simulink library "NelinSys"  (Simulink 2.20)
values from neighbouring files (symbols this model uses):
  v = menu('EXACT LINEARIZATION (demo simulations)',    'Exact linearization of SISO system',    'Exact linearization of MIMO system',    'System with unstable zero dynamics')    [demos_exakt.m]    (also in demos_fp.m = menu('PHASE PLANE ANALYSIS (demo simulations)',    '2nd-Orde; demos_gs.m = menu('GAIN SCHEDULING (demo simulations)',    'Input and out)
  x1 = x(j)    [fazrov_auton2.m]
  x2 = x(j+1)    [fazrov_auton2.m]    (also in fazrov_typ1.m = get_param(get_param(gcbh,'Parent'),'UserData'))
undefined symbols (not defined in the file or in its folder): sfunvxy
libraries: simulink x5
(part 1 of 2)

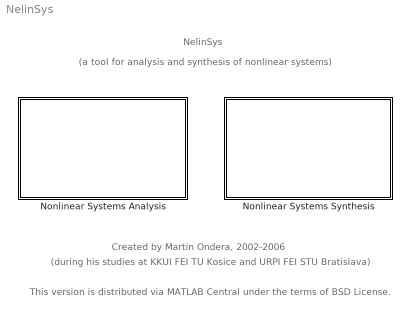
== system NelinSys ==
  note: (a tool for analysis and synthesis of nonlinear systems)
  note: NelinSys
  note: Created by Martin Ondera, 2002-2006
  note: (during his studies at KKUI FEI TU Kosice and URPI FEI STU Bratislava)
  note: This version is distributed via MATLAB Central under the terms of BSD License.
  Nonlinear Systems Analysis : Subsystem
      mask Type: Nonlinear Systems Analysis
      mask Display: disp('Analysis');
  Nonlinear Systems Synthesis : Subsystem
      mask Type: Nonlinear Systems Synthesis
      mask Display: disp('Synthesis');

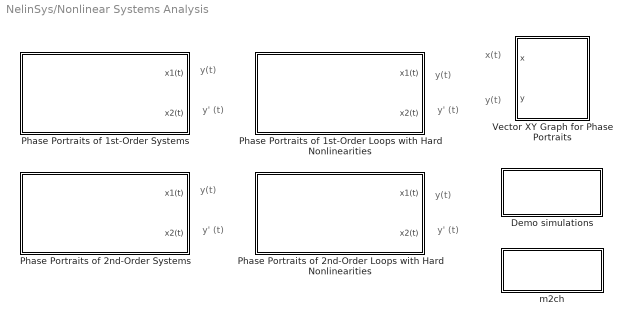
== system NelinSys/Nonlinear Systems Analysis ==
  note: y(t)
  note: y' (t)
  note: x(t)
  note: y(t)
  note: y(t)
  note: y' (t)
  note: y(t)
  note: y' (t)
  note: y(t)
  note: y' (t)
  Demo simulations : Subsystem
      settings: OpenFcn=demos_fp
      mask Display: disp('Phase Plane\nAnalysis')
  Phase Portraits of 1st-Order Loops with Hard Nonlinearities : Subsystem  mask(Phase-Plane Portrait of a 1st-Order Loop with a Hard Nonlinearity){num=0.01, den=[1 0.01], nelintyp=Relay with hysteresis, nelinpar=[-1 0 1 100], w=20, x10=[0 25]}
      mask prompts: num "Linear part - transfer function numerator:"; den "Linear part - transfer function denominator:"; nelintyp "Nonlinear part - nonlinearity type:"; nelinpar "Nonlinear part - parameters:"; w "Setpoint:"; x10 "Initial conditions: x1(0) = y(0) ="
      mask help:
      | Computation of a phase-plane portrait of a closed loop system consisting of an isolated hard nonlinearity and a linear part specified by a 1st-order transfer function.
      |
      | Block has two vector outputs, y = x1 (system output) and y' = x2 (derivative of the system output), i.e. horizontal and vertical coordinates of phase-plane trajectories corresponding to different initial conditions - the initial conditions themselves are specified by the vector x1(0) below.
      |
      | It is recommended to use the "Vector XY Graph for Phase Portraits" block to plot the portrait graphically, since the "XY Graph" block from Sinks library cannot handle vector inputs.
      |
      | For a detailed description of the block, click "Help" button.
      mask init:
      | if (length(den) ~= 2) | (length(num) ~= 1) | (den(1) == 0)
      |     error('Linear part must be a 1st-order system!');
      | end
      | 
      | if (nelintyp == 1) & (length(nelinpar) ~= 2)
      |     error('Invalid number of nonlinearity parameters!');
      | end
      | if (nelintyp > 1) & ((length(nelinpar) ~= 4) | nelinpar(1) > nelinpar(3))
      |     error('Invalid nonlinearity parameters!');
      | end
      | 
      | for k = 1:length(x10)
      |     if (w-x10(k)>nelinpar(1)) & (w-x10(k)<nelinpar(3))
      |         error(['Invalid initial conditions!']);
      |     end
      | end
      mask Help: web(fullfile(cd,'help','fazrov_typ1.html'));
      mask StyleString: edit,edit,popup(Ideal relay|Saturation|Relay with dead-zone|Relay with hysteresis),edit,edit,edit
      mask Display: disp('Phase Portraits of\n1st-Order Loops\nwith Hard Nonlinearities');
  Phase Portraits of 1st-Order Systems : Subsystem  mask(Phase-Plane Portrait of a 1st-Order Autonomous System){vRovnica=Dy-y^2+1=0, x10=[-10 0.9999 (1+1e-6)]}
      mask prompts: vRovnica "System differential equation: y' + f(y) = 0:"; x10 "Initial conditions: y(0) = x1(0) ="
      mask help:
      | Computation of a phase-plane portrait of a 1st-order nonlinear autonomous system. The system is specified by a differential equation y' + f(y) = 0, where y(t) is the output of the system and f(y) is arbitrary continuous function.
      |
      | Block has two vector outputs, y = x1 and y' = x2, i.e. horizontal and vertical coordinates of phase-plane trajectories corresponding to different initial conditions - the initial conditions themselves are specified by the vector x1(0) below.
      |
      | It is recommended to use the "Vector XY Graph for Phase Portraits" block to plot the portrait graphically, since the "XY Graph" block from Sinks library cannot handle vector inputs.
      |
      | For a detailed description of the block, click "Help" button.
      mask init:
      | % Overenie, ci system nie je vyssieho radu %
      | if (~strcmp(findsym(sym(vRovnica)),'Dy, y') & ~strcmp(findsym(sym(vRovnica)),'Dy'))
      | 	error('Error: Invalid differential equation!');
      | end
      | 
      | % Vyjadrenie derivacie vystupu z rovnice %
      | skt = solve(vRovnica, 'Dy');
      mask Help: web(fullfile(cd,'help','fazrov_auton1.html'));
      mask Display: disp('Phase Portraits of 1st-Order\nAutonomous Systems\n\ny'' + f (y) = 0');
  Phase Portraits of 2nd-Order Loops with Hard Nonlinearities : Subsystem  mask(Phase-Plane Portrait of a 2nd-Order Loop with a Hard Nonlinearity){num=1, den=conv([1 3],[1 -1]), nelintyp=Saturation, nelinpar=[-1 -4 1 4], w=0, x1min=-2, x1max=2, x1num=10, x2min=-2, x2max=5, x2num=3}
      mask prompts: num "Linear part - transfer function numerator:"; den "Linear part - transfer function denominator:"; nelintyp "Nonlinear part - nonlinearity type:"; nelinpar "Nonlinear part - parameters:"; w "Setpoint:"; x1min "Initial conditions range: x1(0) minimum"; x1max "Initial conditions range: x1(0) maximum"; x1num "Number of initial conditions for x1"; x2min "Initial conditions range: x2(0) minimum"; x2max "Initial conditions range: x2(0) maximum"; x2num "Number of initial conditions for x2"
      mask help: For a detailed description of block parameters, click "Help" button.
      mask init:
      | if (length(den) ~= 3) | (length(num) ~= 1) | (den(1) == 0)
      |     error('Linear part must be a 2nd-order system!');
      | end
      | 
      | if (nelintyp == 1) & (length(nelinpar) ~= 2)
      |     error('Invalid number of nonlinearity parameters!');
      | end
      | if (nelintyp > 1) & ((length(nelinpar) ~= 4) | nelinpar(1) > nelinpar(3))
      |     error('Invalid nonlinearity parameters!');
      | end
      mask Help: web(fullfile(cd,'help','fazrov_typnl.html'));
      mask StyleString: edit,edit,popup(Ideal relay|Saturation|Relay with dead-zone|Relay with hysteresis),edit,edit,edit,edit,edit,edit,edit,edit
      mask Display: disp('Phase Portraits of\n2nd-Order Loops\nwith Hard Nonlinearities');
  Phase Portraits of 2nd-Order Systems : Subsystem  mask(Phase-Plane Portrait of a 2nd-Order Autonomous System){vRovnica=D2y+(Dy)^2=0, x1min=-5, x1max=5, x1num=10, x2min=-1, x2max=10, x2num=3}
      mask prompts: vRovnica "System differential equation: y'' + f(y, y') = 0:"; x1min "Initial conditions range: y(0) = x1(0) minimum"; x1max "Initial conditions range: y(0) = x1(0) maximum"; x1num "Number of initial conditions for x1"; x2min "Initial conditions range: y' (0) = x2(0) minimum"; x2max "Initial conditions range: y' (0) = x2(0) maximum"; x2num "Number of initial conditions for x2"
      mask help:
      | Computation of a phase-plane portrait of a 2nd-order nonlinear autonomous system. The system is specified by a differential equation y'' + f(y, y') = 0, where y(t) is the output of the system and f(y, y') is arbitrary continuous function.
      |
      | Block has two vector outputs, y = x1 and y' = x2, i.e. horizontal and vertical coordinates of phase-plane trajectories corresponding to different initial conditions - the initial conditions themselves are specified by the range-parameters below.
      |
      | To plot the portrait graphically, it is necessary to use the "Vector XY Graph for Phase Portraits" block, since the "XY Graph" block from Sinks library cannot handle vector inputs.
      |
      | For a detailed description of the block, click "Help" button.
      mask init:
      | % Overenie, ci system nie je vyssieho radu %
      | if (~strcmp(findsym(sym(vRovnica)),'D2y, Dy, y') & ~strcmp(findsym(sym(vRovnica)),'D2y, Dy') & ~strcmp(findsym(sym(vRovnica)),'D2y, y') & ~strcmp(findsym(sym(vRovnica)),'D2y'))
      | 	error('Error: Invalid differential equation!');
      | end
      | 
      | % Vytvorenie kanonickeho tvaru z opisu diferencialnou rovnicou %
      | vRovnica = subs(vRovnica, 'D2y', 'v');
      | vRovnica = subs(vRovnica, 'Dy', 'x2');
      | vRovnica = subs(vRovnica, 'y', 'x1');
      | 
      | % Vyjadrenie druhej derivacie vystupu z rovnice %
      | skt = solve(vRovnica, 'v');
      mask Help: web(fullfile(cd,'help','fazrov_auton2.html'));
      mask Display: disp('Phase Portraits of 2nd-Order\nAutonomous Systems\n\ny'''' + f (y, y'') = 0');
  Vector XY Graph for Phase Portraits : Subsystem  LoadFcn=sfunvxy([],[],[],'LoadBlock')  StartFcn=sfunvxy([],[],[],'Start')  StopFcn=sfunvxy([],[],[],'Stop')  mask(Vector XY Graph for Phase-Plane Portraits){xmin=-6, xmax=6, ymin=-10, ymax=10, st=-1, use_grid=on}
      mask prompts: xmin "x-min:"; xmax "x-max:"; ymin "y-min:"; ymax "y-max:"; st "Sample time (-1 for unspecified):"; use_grid "Show grid"
      mask help:
      | Plots function dependancies of the type Y = Y(X), where X and Y are vectors of the same size (N). In every time instant, N scalar dependancies of the type yi = yi(xi) are plotted simultaneously.
      |
      | The most typical use of the block is to plot phase-plane portraits of systems in which every phase trajectory (every pair of initial conditions) corresponds with one pair of elements of vectors X, Y.
      |
      | For a detailed description of the block, click "Help" button.
      mask init:
      | if (xmin >= xmax) | (ymin >= ymax)
      |     error('Invalid scaling! Must be: x-min < x-max, y-min < y-max.');
      | end
      settings: CopyFcn=sfunvxy([],[],[],'CopyBlock')  DeleteFcn=sfunvxy([],[],[],'DeleteBlock')  NameChangeFcn=sfunvxy([],[],[],'NameChange')
      mask Help: web(fullfile(cd,'help','sfunvxy.html'));
      mask Display:
      | plot([.05 .95 .95 .05 .05],[.45 .45 .95 .95 .45], 0.5+cos(0:0.1:2*pi)*0.3,0.7+sin(0:0.1:2*pi)*0.2)
      | disp('\n\n\nVectorXY')
  m2ch : Subsystem
      settings: OpenFcn=met2char
      mask Display: disp('Two-Characteristics\nMethod')

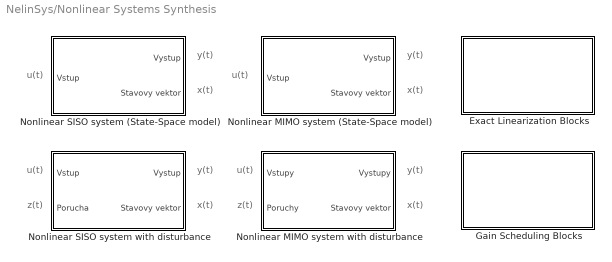
== system NelinSys/Nonlinear Systems Synthesis ==
  note: u(t)
  note: y(t)
  note: x(t)
  note: u(t)
  note: y(t)
  note: x(t)
  note: y(t)
  note: x(t)
  note: y(t)
  note: x(t)
  note: u(t)
  note: u(t)
  note: z(t)
  note: z(t)
  Exact Linearization Blocks : Subsystem
      mask Type: Blocks for Exact Linearization
      mask Display: disp('Exact Linearization');
  Gain Scheduling Blocks : Subsystem
      mask Type: Blocks for Gain Scheduling
      mask Display: disp('Gain Scheduling');
  Nonlinear MIMO system (State-Space model) : Subsystem  mask(Nonlinear MIMO system - state-space model){n=3, F=[84.249*x2*x3; -165.8654*x1*x3-62.5*x2; -15.3846*x3], Fp=0, G=[0 0; 2500 0; 0 0.9799], Gp=0, H=[x1; x3], Hp=0, pp=[0; 0; 1e-9]}
      mask prompts: n "System order (number of states, N)"; F "f(x) - symbolic expression:"; Fp "f(x) - variable identifier:"; G "g(x) - symbolic expression:"; Gp "g(x) - variable identifier:"; H "h(x) - symbolic expression:"; Hp "h(x) - variable identifier:"; pp "Initial conditions (initial states):"
      mask help:
      | Nonlinear MIMO system is described by following nonlinear differential equations:
      |                        dx/dt = f(x) + g(x) u
      |                         y = h(x)
      |
      |              states vector:  x = [x1; x2; ...; xN]
      |              system input: u (vector)
      |              system output: y (vector)
      |
      | Parameters f(x), g(x), h(x) can be specified either as a symbolic expression or as an identifier of a symbolic variable.
      |
      | For a detailed description of parameters, click "Help" button.
      mask init:
      | % Overenie spravnosti zadania parametrov bloku %
      | if ~isempty(F) & (Fp == 0)
      |    F = sym(F);
      | elseif isempty(F) & (any(Fp ~= 0))
      |    F = sym(Fp);
      | else
      |    error(['Matrix f(x) unspecified or specified more than once - cannot continue!']);
      | end
      | 
      | if ~isempty(G) & (Gp == 0)
      |    G = sym(G);
      | elseif isempty(G) & (any(Gp ~= 0))
      |    G = sym(Gp);
      | else
      |    error(['Matrix g(x) unspecified or specified more than once - cannot continue!']);
      | end
      | 
      | if ~isempty(H) & (Hp == 0)
      |    H = sym(H);
      | elseif isempty(H) & (any(Hp ~= 0))
      |    H = sym(Hp);
      | else
      |    error(['Matrix h(x) unspecified or specified more than once - cannot continue!']);
      | end
      | 
      | % Zisti si symbolicke premenne, ktore vystupuju vo vyrazoch %
      | premF = strrep(strrep(findsym(sym(F)),', ',''),',',' ');
      | premG = strrep(strrep(findsym(sym(G)),', ',''),',',' ');
      | premH = strrep(strrep(findsym(sym(H)),', ',''),',',' ');
      | 
      | % Premenne x1, x2, ..., xN su korektne, preskoc ich %
      | for k = 1 : n
      |    premF = strrep(premF, sprintf('x%d',k), '');
      |    premG = strrep(premG, sprintf('x%d',k), '');
      |    premH = strrep(premH, sprintf('x%d',k), '');
      | end
      | 
      | % Ak niektory retazec nezostal prazdny, vyhlas chybu %
      | if ~isempty(premF)
      |    error(['Unknown symbol in f(x) expression - cannot continue!']);
      | end
      | if ~isempty(premG)
      |    error(['Unknown symbol in g(x) expression - cannot continue!']);
      | end
      | if ~isempty(premH)
      |    error(['Unknown symbol in h(x) expression - cannot continue!']);
      | end
      | 
      | % Otestovanie spravnosti rozmerov matic F,G,H (podla "n") %
      | if ~all(size(F) == [n,1])
      |    error(['Invalid matrix dimensions: f(x) - cannot continue!']);
      |    return;
      | end
      | 
      | nin = size(G);
      | if (nin(1,1) ~= n)
      |    error(['Invalid matrix dimensions: g(x) - cannot continue!']);
      |    return;
      | end
      | nin = nin(1,2);
      | 
      | nout = size(H);
      | if (nout(1,2) ~= 1)
      |    error(['Invalid matrix dimensions: h(x) - cannot continue!']);
      |    return;
      | end
      | nout = nout(1,1);
      | 
      | % Kontrola vektora pociatocnych podmienok (pociatocnych stavov) %
      | if ~all(size(pp) == [n,1])
      |    error(['Initial conditions vector: invalid dimensions - cannot continue!']);
      |    return;
      | end
      | 
      | % Nahradenie identifikatorov "xI" identifikatormi "x(I)" %
      | co_str = '{''x1'; cim_str = '{''x(1)';
      | 
      | for k = 2 : n
      |     co_str = sprintf('%s'',''x%d', co_str, k);
      |     cim_str = sprintf('%s'',''x(%d)', cim_str, k);
      | end
      | 
      | co_str = strcat(co_str, '''}'); cim_str = strcat(cim_str, '''}');
      | 
      | F = eval(sprintf('subs(F,%s,%s)', co_str, cim_str));
      | G = eval(sprintf('subs(G,%s,%s)', co_str, cim_str));
      | H = eval(sprintf('subs(H,%s,%s)', co_str, cim_str));
      mask Help: web(fullfile(cd,'help','stavp_mimo.html'));
      mask Display: disp('Nonlinear MIMO system\n\nx'' = f(x) + g(x) u\ny = h(x)');
  Nonlinear MIMO system with disturbance : Subsystem  mask(Nonlinear MIMO system with disturbance - state-space model){n=3, F=[84.249*x2*x3; -165.8654*x1*x3-62.5*x2; -15.3846*x3], Fp=0, G=[0 0; 2500 0; 0 0.9799], Gp=0, H=[x1; x3], Hp=0, E=[-31.746*z1; 0; 0], Ep=0, pp=[0; 0; 1e-9]}
      mask prompts: n "System order (number of states, N)"; F "f(x) - symbolic expression:"; Fp "f(x) - variable identifier:"; G "g(x) - symbolic expression:"; Gp "g(x) - variable identifier:"; H "h(x) - symbolic expression:"; Hp "h(x) - variable identifier:"; E "e(z) - symbolic expression:"; Ep "e(z) - variable identifier:"; pp "Initial conditions (initial states):"
      mask help:
      | Nonlinear MIMO system is described by following nonlinear differential equations:
      |                         dx/dt = f(x) + g(x) u + e(z)
      |                          y = h(x)
      |
      |              states vector:  x = [x1; x2; ...; xN]
      |              disturbances: z = [z1; z2; ... zN]
      |              system inputs: u (vector)
      |              system outputs: y (vector)
      |
      | Parameters f(x), g(x), h(x), e(z) can be specified either as a symbolic expression or as an identifier of a symbolic variable.
      |
      | For a detailed description of parameters, click "Help" button.
      mask init:
      | % Overenie spravnosti zadania parametrov bloku %
      | if ~isempty(F) & (Fp == 0)
      |    F = sym(F);
      | elseif isempty(F) & (any(Fp ~= 0))
      |    F = sym(Fp);
      | else
      |    error(['Matrix f(x) unspecified or specified more than once - cannot continue!']);
      | end
      | 
      | if ~isempty(G) & (Gp == 0)
      |    G = sym(G);
      | elseif isempty(G) & (any(Gp ~= 0))
      |    G = sym(Gp);
      | else
      |    error(['Matrix g(x) unspecified or specified more than once - cannot continue!']);
      | end
      | 
      | if ~isempty(H) & (Hp == 0)
      |    H = sym(H);
      | elseif isempty(H) & (any(Hp ~= 0))
      |    H = sym(Hp);
      | else
      |    error(['Matrix h(x) unspecified or specified more than once - cannot continue!']);
      | end
      | 
      | if ~isempty(E) & (Ep == 0)
      |    E = sym(E);
      | elseif isempty(E) & (any(Ep ~= 0))
      |    E = sym(Ep);
      | else
      |    error(['Matrix e(z) unspecified or specified more than once - cannot continue!']);
      | end
      | 
      | % Zisti si symbolicke premenne, ktore vystupuju vo vyrazoch %
      | premF = strrep(strrep(findsym(sym(F)),', ',''),',',' ');
      | premG = strrep(strrep(findsym(sym(G)),', ',''),',',' ');
      | premH = strrep(strrep(findsym(sym(H)),', ',''),',',' ');
      | premE = strrep(strrep(findsym(sym(E)),', ',''),',',' ');
      | 
      | % Premenne x1, x2, ..., xN su korektne, preskoc ich %
      | for k = 1 : n
      |    premF = strrep(premF, sprintf('x%d',k), '');
      |    premG = strrep(premG, sprintf('x%d',k), '');
      |    premH = strrep(premH, sprintf('x%d',k), '');
      |    premE = strrep(premE, sprintf('z%d',k), '');
      | end
      | 
      | % Ak niektory retazec nezostal prazdny, vyhlas chybu %
      | if ~isempty(premF)
      |    error(['Unknown symbol in f(x) expression - cannot continue!']);
      | end
      | if ~isempty(premG)
      |    error(['Unknown symbol in g(x) expression - cannot continue!']);
      | end
      | if ~isempty(premH)
      |    error(['Unknown symbol in h(x) expression - cannot continue!']);
      | end
      | if ~isempty(premE)
      |    error(['Unknown symbol in e(z) expression - cannot continue!']);
      | end
      | 
      | % Otestovanie spravnosti rozmerov matic F,G,H,E (podla "n") %
      | if ~all(size(sym(F)) == [n,1])
      |    error(['Invalid matrix dimensions: f(x) - cannot continue!']);
      | end
      | 
      | % Zistenie poctu vstupov systemu podla rozmeru G %
      | nin = size(sym(G));
      | if (nin(1,1) ~= n)
      |    error(['Invalid matrix dimensions: g(x) - cannot continue!']);
      | end
      | nin = nin(1,2);
      | 
      | % Zistenie poctu vystupov systemu podla rozmeru H %
      | nout = size(sym(H));
      | if (nout(1,2) ~= 1)
      |    error(['Invalid matrix dimensions: h(x) - cannot continue!']);
      | end
      | nout = nout(1,1);
      | 
      | % Zistenie poctu poruch podla rozmeru E %
      | nz = size(sym(E));
      | if (nz(1,1) ~= n)
      |    error(['Invalid matrix dimensions: e(z) - cannot continue!']);
      | end
      | nz = nz(1,2);
      | 
      | % Kontrola vektora pociatocnych podmienok (pociatocnych stavov) %
      | if ~all(size(pp) == [n,1])
      |    error(['Initial conditions vector: invalid dimensions - cannot continue!']);
      | end
      | 
      | % Nahradenie identifikatorov "xI" identifikatormi "x(I)" %
      | co_str = '{''x1'; cim_str = '{''x(1)';
      | 
      | for k = 2 : n
      |     co_str = sprintf('%s'',''x%d', co_str, k);
      |     cim_str = sprintf('%s'',''x(%d)', cim_str, k);
      | end
      | 
      | co_str = strcat(co_str, '''}'); cim_str = strcat(cim_str, '''}');
      | 
      | F = eval(sprintf('subs(F,%s,%s)', co_str, cim_str));
      | G = eval(sprintf('subs(G,%s,%s)', co_str, cim_str));
      | H = eval(sprintf('subs(H,%s,%s)', co_str, cim_str));
      | 
      | % Nahradenie identifikatorov "zI" identifikatormi "u(nin+I)" %
      | co_str = '{''z1'; cim_str = sprintf('{''u(%d)', nin+1);
      | 
      | for k = 2 : nz
      |    co_str = sprintf('%s'',''z%d', co_str, k);
      |    cim_str = sprintf('%s'',''u(%d)', cim_str, nin+k);
      | end
      | 
      | co_str = strcat(co_str, '''}'); cim_str = strcat(cim_str, '''}');
      | E = eval(sprintf('subs(E,%s,%s)', co_str, cim_str));
      mask Help: web(fullfile(cd,'help','stavp_mimoz.html'));
      mask Display: disp('Nonlinear MIMO system\nwith disturbance\n\nx'' = f(x) + g(x) u + e(z)\ny = h(x)');
  Nonlinear SISO system (State-Space model) : Subsystem  mask(Nonlinear SISO system - state-space model){n=2, F=[-sqrt(x1); sqrt(x1)-sqrt(x2)], Fp=0, G=[1; 0], Gp=0, H=x2, Hp=0, pp=[0.1; 0.01]}
      mask prompts: n "System order (number of states, N)"; F "f(x) - symbolic expression:"; Fp "f(x) - variable identifier:"; G "g(x) - symbolic expression:"; Gp "g(x) - variable identifier:"; H "h(x) - symbolic expression:"; Hp "h(x) - variable identifier:"; pp "Initial conditions (initial states):"
      mask help:
      | Nonlinear SISO system is described by following nonlinear differential equations:
      |                      dx/dt = f(x) + g(x) u
      |                       y = h(x)
      |
      |              states vector:  x = [x1; x2; ...; xN]
      |              system input: u
      |              system output: y
      |
      | Parameters f(x), g(x), h(x) can be specified either as a symbolic expression or as an identifier of a symbolic variable.
      |
      | For a detailed description of parameters, click "Help" button.
      mask init:
      | % Overenie spravnosti zadania parametrov bloku %
      | if ~isempty(F) & (Fp == 0)
      |    F = sym(F);
      | elseif isempty(F) & (any(Fp ~= 0))
      |    F = sym(Fp);
      | else
      |    error(['Matrix f(x) unspecified or specified more than once - cannot continue!']);
      | end
      | 
      | if ~isempty(G) & (Gp == 0)
      |    G = sym(G);
      | elseif isempty(G) & (any(Gp ~= 0))
      |    G = sym(Gp);
      | else
      |    error(['Matrix g(x) unspecified or specified more than once - cannot continue!']);
      | end
      | 
      | if ~isempty(H) & (Hp == 0)
      |    H = sym(H);
      | elseif isempty(H) & (any(Hp ~= 0))
      |    H = sym(Hp);
      | else
      |    error(['Matrix h(x) unspecified or specified more than once - cannot continue!']);
      | end
      | 
      | % Zisti si symbolicke premenne, ktore vystupuju vo vyrazoch %
      | premF = strrep(strrep(findsym(sym(F)),', ',''),',',' ');
      | premG = strrep(strrep(findsym(sym(G)),', ',''),',',' ');
      | premH = strrep(strrep(findsym(sym(H)),', ',''),',',' ');
      | 
      | % Premenne x1, x2, ..., xN su korektne, preskoc ich %
      | for k = 1 : n
      |    premF = strrep(premF, sprintf('x%d',k), '');
      |    premG = strrep(premG, sprintf('x%d',k), '');
      |    premH = strrep(premH, sprintf('x%d',k), '');
      | end
      | 
      | % Ak niektory retazec nezostal prazdny, vyhlas chybu %
      | if ~isempty(premF)
      |    error(['Unknown symbol in f(x) expression - cannot continue!']);
      | end
      | if ~isempty(premG)
      |    error(['Unknown symbol in g(x) expression - cannot continue!']);
      | end
      | if ~isempty(premH)
      |    error(['Unknown symbol in h(x) expression - cannot continue!']);
      | end
      | 
      | % Otestovanie spravnosti rozmerov matic F,G,H (podla "n") %
      | if ~all(size(F) == [n,1])
      |    error(['Invalid matrix dimensions: f(x) - cannot continue!']);
      | end
      | if ~all(size(G) == [n,1])
      |    error(['Invalid matrix dimensions: g(x) - cannot continue!']);
      | end
      | if ~all(size(H) == [1,1])
      |    error(['Invalid matrix dimensions: h(x) - cannot continue!']);
      | end
      | 
      | % Kontrola vektora pociatocnych podmienok (pociatocnych stavov) %
      | if ~all(size(pp) == [n,1])
      |    error(['Invalid dimensions: initial conditions vector - cannot continue!']);
      | end
      | 
      | % Nahradenie identifikatorov "xI" identifikatormi "x(I)" %
      | co_str = '{''x1'; cim_str = '{''x(1)';
      | 
      | for k = 2 : n
      |     co_str = sprintf('%s'',''x%d', co_str, k);
      |     cim_str = sprintf('%s'',''x(%d)', cim_str, k);
      | end
      | 
      | co_str = strcat(co_str, '''}'); cim_str = strcat(cim_str, '''}');
      | 
      | F = eval(sprintf('subs(F,%s,%s)', co_str, cim_str));
      | G = eval(sprintf('subs(G,%s,%s)', co_str, cim_str));
      | H = eval(sprintf('subs(H,%s,%s)', co_str, cim_str));
      mask Help: web(fullfile(cd,'help','stavp_siso.html'));
      mask Display: disp('Nonlinear SISO system\n\nx'' = f(x) + g(x) u\ny = h(x)');
  Nonlinear SISO system with disturbance : Subsystem  mask(Nonlinear SISO system with disturbance - state-space model){n=2, F=[-sqrt(x1); sqrt(x1)-sqrt(x2)], Fp=0, G=[1; 0], Gp=0, H=x2, Hp=0, E=[z; 0], Ep=0, pp=[0.1; 0.01]}
      mask prompts: n "System order (number of states, N)"; F "f(x) - symbolic expression:"; Fp "f(x) - variable identifier:"; G "g(x) - symbolic expression:"; Gp "g(x) - variable identifier:"; H "h(x) - symbolic expression:"; Hp "h(x) - variable identifier:"; E "e(z) - symbolic expression:"; Ep "e(z) - variable identifier:"; pp "Initial conditions (initial states):"
      mask help:
      | Nonlinear SISO system is described by following nonlinear differential equations:
      |                       dx/dt = f(x) + g(x) u + e(z)
      |                        y = h(x)
      |
      |              states vector:  x = [x1; x2; ...; xN]
      |              system input: u
      |              system output: y
      |              disturbance: z
      |
      | Parameters f(x), g(x), h(x), e(z) can be specified either as a symbolic expression or as an identifier of a symbolic variable.
      |
      | For a detailed description of parameters, click "Help" button.
      mask init:
      | % Overenie spravnosti zadania parametrov bloku %
      | if ~isempty(F) & (Fp == 0)
      |    F = sym(F);
      | elseif isempty(F) & (any(Fp ~= 0))
      |    F = sym(Fp);
      | else
      |    error(['Matrix f(x) unspecified or specified more than once - cannot continue!']);
      | end
      | 
      | if ~isempty(G) & (Gp == 0)
      |    G = sym(G);
      | elseif isempty(G) & (any(Gp ~= 0))
      |    G = sym(Gp);
      | else
      |    error(['Matrix g(x) unspecified or specified more than once - cannot continue!']);
      | end
      | 
      | if ~isempty(H) & (Hp == 0)
      |    H = sym(H);
      | elseif isempty(H) & (any(Hp ~= 0))
      |    H = sym(Hp);
      | else
      |    error(['Matrix h(x) unspecified or specified more than once - cannot continue!']);
      | end
      | 
      | if ~isempty(E) & (Ep == 0)
      |    E = sym(E);
      | elseif isempty(E) & (any(Ep ~= 0))
      |    E = sym(Ep);
      | else
      |    error(['Matrix e(z) unspecified or specified more than once - cannot continue!']);
      | end
      | 
      | % Zisti si symbolicke premenne, ktore vystupuju vo vyrazoch %
      | premF = strrep(strrep(findsym(sym(F)),', ',''),',',' ');
      | premG = strrep(strrep(findsym(sym(G)),', ',''),',',' ');
      | premH = strrep(strrep(findsym(sym(H)),', ',''),',',' ');
      | premE = strrep(strrep(findsym(sym(E)),', ',''),',',' ');
      | 
      | % Premenne x1, x2, ..., xN su korektne, preskoc ich %
      | for k = 1 : n
      |    premF = strrep(premF, sprintf('x%d',k), '');
      |    premG = strrep(premG, sprintf('x%d',k), '');
      |    premH = strrep(premH, sprintf('x%d',k), '');
      | end
      | 
      | % Ak niektory retazec nezostal prazdny, vyhlas chybu %
      | if ~isempty(premF)
      |    error(['Unknown symbol in f(x) expression - cannot continue!']);
      | end
      | if ~isempty(premG)
      |    error(['Unknown symbol in g(x) expression - cannot continue!']);
      | end
      | if ~isempty(premH)
      |    error(['Unknown symbol in h(x) expression - cannot continue!']);
      | end
      | if ~isempty(premE) & ~strcmp(premE,'z')
      |    error(['Unknown symbol in e(z) expression - cannot continue!']);
      | end
      | 
      | % Otestovanie spravnosti rozmerov matic F,G,H,E (podla "n") %
      | if ~all(size(sym(F)) == [n,1])
      |    error(['Invalid matrix dimensions: f(x) - cannot continue!']);
      | end
      | if ~all(size(sym(G)) == [n,1])
      |    error(['Invalid matrix dimensions: g(x) - cannot continue!']);
      | end
      | if ~all(size(sym(E)) == [n,1])
      |    error(['Invalid matrix dimensions: e(z) - cannot continue!']);
      | end
      | if ~all(size(sym(H)) == [1,1])
      |    error(['Invalid matrix dimensions: h(x) - cannot continue!']);
      | end
      | 
      | % Kontrola vektora pociatocnych podmienok (pociatocnych stavov) %
      | if ~all(size(pp) == [n,1])
      |    error(['Initial conditions vector: invalid dimensions - cannot continue!']);
      | end
      | 
      | % Nahradenie identifikatorov "xI" identifikatormi "x(I)" %
      | co_str = '{''x1'; cim_str = '{''x(1)';
      | 
      | for k = 2 : n
      |     co_str = sprintf('%s'',''x%d', co_str, k);
      |     cim_str = sprintf('%s'',''x(%d)', cim_str, k);
      | end
      | 
      | co_str = strcat(co_str, '''}'); cim_str = strcat(cim_str, '''}');
      | 
      | F = eval(sprintf('subs(F,%s,%s)', co_str, cim_str));
      | G = eval(sprintf('subs(G,%s,%s)', co_str, cim_str));
      | H = eval(sprintf('subs(H,%s,%s)', co_str, cim_str));
      | 
      | % Nahradenie identifikatora "z" identifikatorom "u(2)" %
      | E = subs(E, 'z','u(2)');
      mask Help: web(fullfile(cd,'help','stavp_sisoz.html'));
      mask Display: disp('Nonlinear SISO system\nwith disturbance\n\nx'' = f(x) + g(x) u + e(z)\ny = h(x)');

== system NelinSys/Nonlinear Systems Analysis/Demo simulations ==

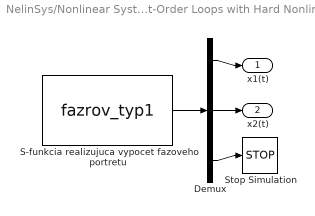
== system NelinSys/Nonlinear Systems Analysis/Phase Portraits of 1st-Order Loops with Hard Nonlinearities ==
  Demux : Demux  Outputs=[length(x10) length(x10) 1]
  S-funkcia realizujuca vypocet fazoveho portretu : S-Function  FunctionName=fazrov_typ1  Parameters=num,den,w,nelintyp,nelinpar,x10  PortCounts=[]  SFunctionModules=''
  Stop Simulation : Stop
  x1(t) : Outport  Port=1
  x2(t) : Outport  Port=2
  wires:
  Demux/1 -> x1(t)/1
  S-funkcia realizujuca vypocet fazoveho portretu/1 -> Demux/1
  Demux/2 -> x2(t)/1
  Demux/3 -> Stop Simulation/1

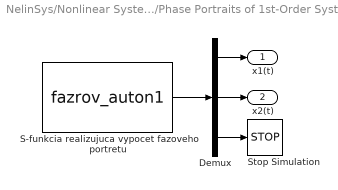
== system NelinSys/Nonlinear Systems Analysis/Phase Portraits of 1st-Order Systems ==
  Demux : Demux  Outputs=[length(x10) length(x10) 1]
  S-funkcia realizujuca vypocet fazoveho portretu : S-Function  FunctionName=fazrov_auton1  Parameters=skt,x10  PortCounts=[]  SFunctionModules=''
  Stop Simulation : Stop
  x1(t) : Outport  Port=1
  x2(t) : Outport  Port=2
  wires:
  S-funkcia realizujuca vypocet fazoveho portretu/1 -> Demux/1
  Demux/1 -> x1(t)/1
  Demux/2 -> x2(t)/1
  Demux/3 -> Stop Simulation/1

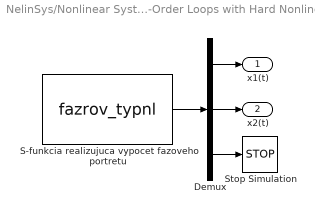
== system NelinSys/Nonlinear Systems Analysis/Phase Portraits of 2nd-Order Loops with Hard Nonlinearities ==
  Demux : Demux  Outputs=[(x1num*x2num) (x1num*x2num) 1]
  S-funkcia realizujuca vypocet fazoveho portretu : S-Function  FunctionName=fazrov_typnl  Parameters=num,den,w,nelintyp,nelinpar,x1min,x1max,x1num,x2min,x2max,x2num  PortCounts=[]  SFunctionModules=''
  Stop Simulation : Stop
  x1(t) : Outport  Port=1
  x2(t) : Outport  Port=2
  wires:
  Demux/2 -> x2(t)/1
  S-funkcia realizujuca vypocet fazoveho portretu/1 -> Demux/1
  Demux/1 -> x1(t)/1
  Demux/3 -> Stop Simulation/1

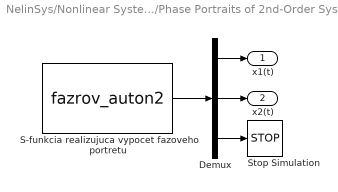
== system NelinSys/Nonlinear Systems Analysis/Phase Portraits of 2nd-Order Systems ==
  Demux : Demux  Outputs=[(x1num*x2num) (x1num*x2num) 1]
  S-funkcia realizujuca vypocet fazoveho portretu : S-Function  FunctionName=fazrov_auton2  Parameters=skt,x1min,x1max,x1num,x2min,x2max,x2num  PortCounts=[]  SFunctionModules=''
  Stop Simulation : Stop
  x1(t) : Outport  Port=1
  x2(t) : Outport  Port=2
  wires:
  S-funkcia realizujuca vypocet fazoveho portretu/1 -> Demux/1
  Demux/1 -> x1(t)/1
  Demux/2 -> x2(t)/1
  Demux/3 -> Stop Simulation/1

== system NelinSys/Nonlinear Systems Analysis/Vector XY Graph for Phase Portraits ==
  x : Inport  Port=1  PortWidth=-1  SampleTime=-1
  y : Inport  Port=2  PortWidth=-1  SampleTime=-1
  Mux : Mux  Inputs=2
  sfunvxy : S-Function  FunctionName=sfunvxy  Parameters=[xmin xmax ymin ymax],use_grid,st  PortCounts=[]  SFunctionModules=''
  wires:
  y/1 -> Mux/2
  x/1 -> Mux/1
  Mux/1 -> sfunvxy/1

== system NelinSys/Nonlinear Systems Analysis/m2ch ==

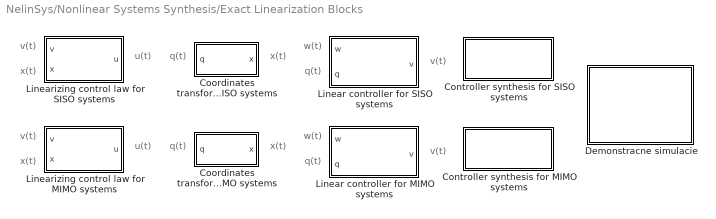
== system NelinSys/Nonlinear Systems Synthesis/Exact Linearization Blocks ==
  note: x(t)
  note: x(t)
  note: q(t)
  note: q(t)
  note: u(t)
  note: u(t)
  note: v(t)
  note: x(t)
  note: v(t)
  note: x(t)
  note: w(t)
  note: q(t)
  note: v(t)
  note: w(t)
  note: q(t)
  note: v(t)
  Controller synthesis for MIMO systems : Subsystem
      settings: OpenFcn=exaktmimo
      mask Type: Exact linearization for MIMO systems
      mask Display: disp('ExactMIMO');
  Controller synthesis for SISO systems : Subsystem
      settings: OpenFcn=exaktsiso
      mask Type: Exact linearization for SISO systems
      mask Display: disp('ExactSISO');
  Coordinates transformation for MIMO systems : Subsystem  Orientation=left  mask(Coordinates transformation for MIMO systems){n=3, r=[2 1], Z=[x1; 84.249*x2*x3; x3], Zp=0}
      mask prompts: n "System order (number of states, N):"; r "Relative degrees of subsystems (r1+r2+...+rK <= n):"; Z "Transformation formula - symbolic expression: q = Q(x) ="; Zp "Transformation formula - variable identifier:"
      mask help:
      | This block performs a nonlinear transformation of system state variables according to the exact linearization rules. Together with the corresponding "Linearizing control law" block, it implements a transformation
      |
      |                dx/dt = f(x) + g(x) u          --->          dq/dt = Aq + Bv
      |                       y = h(x)                     --->                 y = Cq
      |
      | i.e. the transformation of a nonlinear system into a linear and controllable form. This version of the block is designed for use with MIMO systems. To compute the coordinates transformation Q = Q(x) for a given system, the "ExaktMimo.m" application can be used.
      |
      | Transformation formula can be specified either as a symbolic expression or as an identifier of a symbolic variable.
      |
      | For a detailed description of block parameters, click "Help" button below.
      mask init:
      | % Overenie spravnosti zadania parametrov bloku %
      | if ~isempty(Z) & (Zp == 0)
      |    Z = sym(Z);
      | elseif isempty(Z) & (any(Zp ~= 0))
      |    Z = sym(Zp);
      | else
      |    error(['Transformation formula not specified or specified more than once - cannot continue!']);
      | end
      | 
      | % Zisti si symbolicke premenne, ktore vystupuju vo vyraze %
      | prem = strrep(strrep(findsym(sym(Z)),', ',''),',',' ');
      | 
      | % Premenne x1, x2, ..., xN su korektne, preskoc ich %
      | for k = 1 : n
      |    prem = strrep(prem, sprintf('x%d',k), '');
      | end
      | 
      | % Ak retazec nezostal prazdny, vyhlas chybu %
      | if ~isempty(prem)
      |    error(['Unknown symbol found in transformation formula - cannot continue!']);
      | end
      | 
      | if (sum(r) > n)
      |  error('Error: Total relative degree (i.e. the sum of relative degrees of subsystems) cannot be higher than system order!');
      | end
      | 
      | % Otestovanie spravnosti rozmeru matice Z (podla "r") %
      | if ~all(size(sym(Z)) == [sum(r),1])
      |    error(['Wrong number of transformation equations (wrong number of rows of transformation matrix) !']);
      | end
      | 
      | % Nahradenie identifikatorov "xI" identifikatormi "u(I)" %
      | co_str = '{''x1'; cim_str = '{''u(1)';
      | 
      | for k = 2 : n
      |     co_str = sprintf('%s'',''x%d', co_str, k);
      |     cim_str = sprintf('%s'',''u(%d)', cim_str, k);
      | end
      | 
      | co_str = strcat(co_str, '''}'); cim_str = strcat(cim_str, '''}');
      | Z = eval(sprintf('subs(Z,%s,%s)', co_str, cim_str));
      mask Help: web(fullfile(cd,'help','transf_mimo.html'));
      mask Display: disp('Q = Q(X)');
  Coordinates transformation for SISO systems : Subsystem  Orientation=left  mask(Coordinates transformation for SISO systems){n=2, r=2, Z=[x2; sqrt(x1)-sqrt(x2)], Zp=0}
      mask prompts: n "System order (number of states, N):"; r "Relative degree of the system (r <= n):"; Z "Transformation formula - symbolic expression: q = q(x) ="; Zp "Transformation formula - variable identifier:"
      mask help:
      | This block performs a nonlinear transformation of system state variables according to the exact linearization rules. Together with the corresponding "Linearizing control law" block, it implements a transformation
      |
      |                dx/dt = f(x) + g(x) u          --->          dq/dt = Aq + bv
      |                       y = h(x)                     --->                 y = cq
      |
      | i.e. the transformation of a nonlinear system into a linear and controllable form. This version of the block is designed for use with SISO systems. To compute the coordinates transformation q = q(x) for a given system, the "Exakt.m" application can be used.
      |
      | Transformation formula can be specified either as a symbolic expression or as an identifier of a symbolic variable.
      |
      | For a detailed description of block parameters, click "Help" button below.
      mask init:
      | % Overenie spravnosti zadania parametrov bloku %
      | if ~isempty(Z) & (Zp == 0)
      |    Z = sym(Z);
      | elseif isempty(Z) & (any(Zp ~= 0))
      |    Z = Zp;
      | else
      |    error(['Transformation formula not specified or specified more than once - cannot continue!']);
      | end
      | 
      | % Zisti si symbolicke premenne, ktore vystupuju vo vyraze %
      | prem = strrep(strrep(findsym(sym(Z)),', ',''),',',' ');
      | 
      | % Premenne x1, x2, ..., xN su korektne, preskoc ich %
      | for k = 1 : n
      |    prem = strrep(prem, sprintf('x%d',k), '');
      | end
      | 
      | % Ak retazec nezostal prazdny, vyhlas chybu %
      | if ~isempty(prem)
      |    error(['Unknown symbol found in transformation formula - cannot continue!']);
      | end
      | 
      | if (r > n)
      |  error('Error: Relative degree cannot be higher than system order!');
      | end
      | 
      | % Otestovanie spravnosti rozmeru matice Z (podla "r") %
      | if ~all(size(sym(Z)) == [r,1])
      |    error(['Wrong number of transformation equations!']);
      | end
      | 
      | % Nahradenie identifikatorov "xI" identifikatormi "u(I)" %
      | co_str = '{''x1'; cim_str = '{''u(1)';
      | 
      | for k = 2 : n
      |     co_str = sprintf('%s'',''x%d', co_str, k);
      |     cim_str = sprintf('%s'',''u(%d)', cim_str, k);
      | end
      | 
      | co_str = strcat(co_str, '''}'); cim_str = strcat(cim_str, '''}');
      | Z = eval(sprintf('subs(Z,%s,%s)', co_str, cim_str));
      mask Help: web(fullfile(cd,'help','transf_surad.html'));
      mask Display: disp('q = q(x)');
  Demonstracne simulacie : Subsystem
      settings: OpenFcn=demos_exakt
      mask Display: disp('Demo\nsimulations')
  Linear controller for MIMO systems : Subsystem  mask(State-space controller for an integrator-type MIMO system){r=[2 1], nout=2, kor=[-20 -20 -20], integ=off}
      mask prompts: r "Orders of subsystems of the linear MIMO system:"; nout "Number of inputs/outputs of the system:"; kor "Desired poles of a closed-loop system:"; integ "Controller includes integral actions (one per each subsystem)"
      mask help:
      | This block works as a linear state-space controller for MIMO systems with autonomous subsystems of "rI-integrator" type described by state-space equations in a so-called 1st Frobenius form (see help for details). Controller is calculated via pole placement technique during block initialization. Block is typically used in exact-linearization-based control loops.
      |
      | Important: This controller is intended ONLY to control linear MIMO systems of the structure described above and does not work correctly with any other systems!
      |
      | For a detailed description of block parameters, click "Help" button below.
      mask init:
      | if ~all(r>0)
      |    error('Linear controller: Invalid subsytem orders!');
      | end
      | if (nout<0)
      |    error('Linear controller: Wrong number of inputs/outputs!');
      | end
      | if (size(r)~=[nout,1]) & (size(r)~=[1,nout])
      |    error('Linear controller: Number of subsystems not corresponding with the number of inputs/outputs!');
      | end
      | if (length(kor) ~= sum(r)+nout*integ)
      |    error('Linear controller: Wrong number of desired poles!');
      | end
      | 
      | C = zeros(nout,sum(r));
      | K = zeros(nout,sum(r));
      | Ki = zeros(nout,1);
      | P = zeros(nout,1);
      | 
      | i1 = 1;
      | i2 = 1;
      | for l = 1 : nout
      | 
      |    char_polynom = poly(kor(i1:i1+r(l)+integ-1));
      |    K(l,i2:i2+r(l)-1) = fliplr(char_polynom(2:r(l)+1));
      |    C(l,i2) = 1;
      | 
      |    if (integ)
      |       Ki(l) = char_polynom(r(l)+2);
      |       P(l) = 0;
      |    else
      |       Ki(l) = 0;
      |       P(l) = char_polynom(end);
      |    end
      | 
      |    i1 = i1+r(l)+integ;
      |    i2 = i2+r(l);
      | end
      | 
      | Ki = diag(Ki);
      | P = diag(P);
      mask Help: web(fullfile(cd,'help','ppreg_mimo.html'));
      mask Display: disp('Pole Placement\nMIMO');
  Linear controller for SISO systems : Subsystem  mask(State-space controller for an "r-integrator" SISO system){r=2, kor=[-2 -2], integ=off}
      mask prompts: r "Linear system order:"; kor "Desired poles of a closed-loop system:"; integ "Controller includes integral action"
      mask help:
      | This block works as a linear state-space controller for an "r-integrator" SISO system in a so-called 1st Frobenius form (see help for details). Controller is calculated via pole placement technique during block initialization. Block is typically used in exact-linearization-based control loops.
      |
      | Important: This controller is intended ONLY to control linear "r-integrator" SISO systems in 1st Frobenius form and does not work correctly with any other systems!
      |
      | For a detailed description of block parameters, click "Help" button below.
      mask init:
      | if (length(kor) ~= r+integ)
      | 	error('Linear controller: Wrong number of desired poles');
      | end
      | 
      | char_polynom = poly(kor);
      | K = fliplr(char_polynom(2:r+1));
      | 
      | if (integ)
      | 	Ki =char_polynom(r+2);
      | else
      | 	Ki = 0;
      | end
      mask Help: web(fullfile(cd,'help','ppreg_siso.html'));
      mask Display: disp('Pole Placement\nSISO');
  Linearizing control law for MIMO systems : Subsystem  mask(Linearizing control law for MIMO systems){n=3, nout=2, vzorec=[1167173990052591/17592186044416000*x1*x3+1/40*x2+2/421245/x3*v1-1/2500*x2/x3*v2; 153846/9799*x3+10000/9799*v2], vzorecP=0}
      mask prompts: n "System order (number of states, N)"; nout "Number of system outputs:"; vzorec "Linearizing law - symbolic expression: u = U(x,v) ="; vzorecP "Linearizing law - variable identifier:"
      mask help:
      | This block performs a feedback compensation of system nonlinearities according to the exact linearization rules. Together with the "Coordinates transformation" block, it implements a transformation
      |
      |                dx/dt = f(x) + g(x) u          --->          dq/dt = Aq + bv
      |                       y = h(x)                     --->                 y = cq
      |
      | i.e. the transformation of a nonlinear system into a linear and controllable form. This version of the block is designed for use with MIMO systems. To compute the linearization control law U = U(X,V) for a given system, the "ExaktMimo.m" application can be used.
      |
      | Linearizing control law can be specified either as a symbolic expression or as an identifier of a symbolic variable.
      |
      | For a detailed description of block parameters, click "Help" button below.
      mask init:
      | % Overenie spravnosti zadania parametrov bloku %
      | if ~isempty(vzorec) & (vzorecP == 0)
      |    vzorec = sym(vzorec);
      | elseif isempty(vzorec) & (any(vzorecP ~= 0))
      |    vzorec = sym(vzorecP);
      | else
      |    error(['Linearizing law not specified or specified more than once - cannot continue!']);
      | end
      | 
      | % Zisti si symbolicke premenne, ktore vystupuju vo vyraze %
      | prem = strrep(strrep(findsym(sym(vzorec)),', ',''),',',' ');
      | 
      | % Premenne x1, x2, ..., xN su korektne, preskoc ich %
      | for k = 1 : n
      |    prem = strrep(prem, sprintf('x%d',k), '');
      | end
      | 
      | % Aj "v" je korektne, preskoc aj to %
      | for k = 1 : nout
      |    prem = strrep(prem, sprintf('v%d',k), '');
      | end
      | 
      | % Ak retazec nezostal prazdny, vyhlas chybu %
      | if ~isempty(prem)
      |    error(['Unknown symbol in the linearizing law - cannot continue!']);
      | end
      | 
      | % Nahradenie identifikatorov "xI" identifikatormi "u(I+nout)" %
      | co_str = '{''x1'; cim_str = sprintf('{''u(%d)',nout+1);
      | 
      | for k = 2 : n
      |     co_str = sprintf('%s'',''x%d', co_str, k);
      |     cim_str = sprintf('%s'',''u(%d)', cim_str, nout+k);
      | end
      | 
      | % Nahradenie identifikatorov "vI" identifikatormi "u(1)" %
      | for k = 1 : nout
      |     co_str = sprintf('%s'',''v%d', co_str, k);
      |     cim_str = sprintf('%s'',''u(%d)', cim_str, k);
      | end
      | 
      | co_str = strcat(co_str, '''}'); cim_str = strcat(cim_str, '''}');
      | vzorec = eval(sprintf('subs(vzorec,%s,%s)', co_str, cim_str));
      mask Help: web(fullfile(cd,'help','lineariz_mimo.html'));
      mask Display: disp('U = U(X,V)');
  Linearizing control law for SISO systems : Subsystem  mask(Linearizing control law for SISO systems){n=2, vzorec=x1/sqrt(x2)+2*sqrt(x1)*v, vzorecP=0}
      mask prompts: n "System order (number of states, N)"; vzorec "Linearizing law - symbolic expression: u = u(x,v) ="; vzorecP "Linearizing law - variable identifier:"
      mask help:
      | This block performs a feedback compensation of system nonlinearities according to the exact linearization rules. Together with the "Coordinates transformation" block, it implements a transformation
      |
      |                dx/dt = f(x) + g(x) u          --->          dq/dt = Aq + bv
      |                       y = h(x)                     --->                 y = cq
      |
      | i.e. the transformation of a nonlinear system into a linear and controllable form. This version of the block is designed for use with SISO systems. To compute the linearization control law u = u(x,v) for a given system, the "Exakt.m" application can be used.
      |
      | Linearizing control law can be specified either as a symbolic expression or as an identifier of a symbolic variable.
      |
      | For a detailed description of block parameters, click "Help" button below.
      mask init:
      | % Overenie spravnosti zadania parametrov bloku %
      | if isempty(n)
      |    error(['System order not specified - cannot continue!']);
      | end
      | 
      | if ~isempty(vzorec) & (vzorecP == 0)
      |    vzorec = sym(vzorec);
      | elseif isempty(vzorec) & (any(vzorecP ~= 0))
      |    vzorec = sym(vzorecP);
      | else
      |    error(['Linearizing law not specified or specified more than once - cannot continue!']);
      | end
      | 
      | % Zisti si symbolicke premenne, ktore vystupuju vo vyraze %
      | prem = strrep(strrep(findsym(sym(vzorec)),', ',''),',',' ');
      | 
      | % Premenne x1, x2, ..., xN su korektne, preskoc ich %
      | for k = 1 : n
      |    prem = strrep(prem, sprintf('x%d',k), '');
      | end
      | 
      | % Aj "v" je korektne, preskoc aj to %
      | prem = strrep(prem,'v','');
      | 
      | % Ak niektory retazec nezostal prazdny, vyhlas chybu %
      | if ~isempty(prem)
      |    error(['Unknown symbol in the linearizing law - cannot continue!']);
      | end
      | 
      | % Nahradenie identifikatorov "xI" identifikatormi "u(I+1)" a "v" pomocou "u(1)" %
      | co_str = '{''v'',''x1'; cim_str = '{''u(1)'',''u(2)';
      | 
      | for k = 2 : n
      |     co_str = sprintf('%s'',''x%d', co_str, k);
      |     cim_str = sprintf('%s'',''u(%d)', cim_str, k+1);
      | end
      | 
      | co_str = strcat(co_str, '''}'); cim_str = strcat(cim_str, '''}');
      | vzorec = eval(sprintf('subs(vzorec,%s,%s)', co_str, cim_str));
      mask Help: web(fullfile(cd,'help','lineariz_vztah.html'));
      mask Display: disp('u = u(x,v)');
